simulink model "Vehicle_Validation"  (R2013a)
settings: Solver=ode45  StartTime=0.0  StopTime=10.0  RelTol=1e-3
values from neighbouring files (symbols this model uses):
  Beta = 0    [Vehicle_Val.m]    (also in Vehicle_Val_coastdown.m)
  ks_cmd = .15    (= 0.15)    [Vehicle_Val.m]    (also in Vehicle_Val_coastdown.m)
  Or = 0    [Vehicle_Val.m]    (also in Vehicle_Val_coastdown.m = -0.0157)
  Rc = 10000    [Vehicle_Val.m]    (also in Vehicle_Val_coastdown.m)
  rho = 1.2    [Vehicle_Val.m]    (also in Vehicle_Val_coastdown.m)
  V_cmd = 40    [Vehicle_Val.m]    (also in Vehicle_Val_coastdown.m = 0)
libraries: simulink x2
settings Model: Creator=Nathan  LastModifiedBy=Nathan
settings SolverCC: ZeroCrossControl=DisableAll

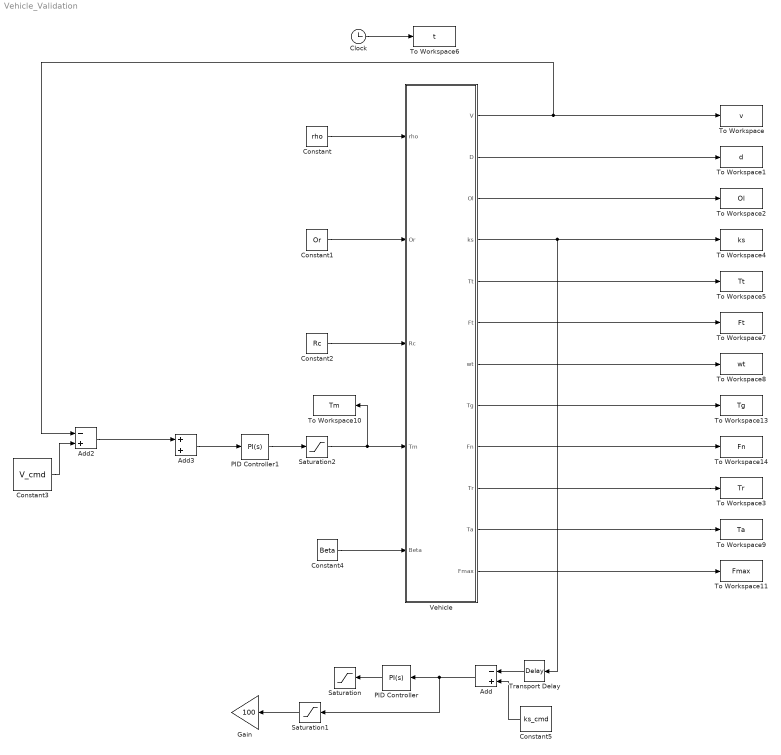
== system Vehicle_Validation ==
  Add : Sum  Inputs=-+
  Add2 : Sum  Inputs=-+
  Add3 : Sum
  Clock : Clock
  Constant : Constant  Value=rho
  Constant1 : Constant  Value=Or
  Constant2 : Constant  Value=Rc
  Constant3 : Constant  Value=V_cmd
  Constant4 : Constant  Value=Beta
  Constant5 : Constant  Value=ks_cmd
  Gain : Gain  Gain=100
  PID Controller : simulink/Continuous/PID Controller  Controller=PI  TimeDomain=Continuous-time  SampleTime=1  IntegratorMethod=Forward Euler  FilterMethod=Forward Euler  Form=Parallel  P=1000  I=5  D=1  N=100  InitialConditionSource=internal  InitialConditionForIntegrator=0  InitialConditionForFilter=0  ExternalReset=none  LimitOutput=off  UpperSaturationLimit=inf  LowerSaturationLimit=-inf  LinearizeAsGain=on  AntiWindupMode=none  Kb=1  TrackingMode=off  Kt=1  PParamMin=[]  PParamMax=[]  IParamMin=[]  IParamMax=[]  DParamMin=[]  DParamMax=[]  NParamMin=[]  NParamMax=[]  KbParamMin=[]  KbParamMax=[]  KtParamMin=[]  KtParamMax=[]  POutMin=[]  POutMax=[]  IOutMin=[]  IOutMax=[]  DOutMin=[]  DOutMax=[]  NOutMin=[]  NOutMax=[]  KbOutMin=[]  KbOutMax=[]  KtOutMin=[]  KtOutMax=[]  IntegratorOutMin=[]  IntegratorOutMax=[]  FilterOutMin=[]  FilterOutMax=[]  SumOutMin=[]  SumOutMax=[]  SumI1OutMin=[]  SumI1OutMax=[]  SumI2OutMin=[]  SumI2OutMax=[]  SumI3OutMin=[]  SumI3OutMax=[]  SumDOutMin=[]  SumDOutMax=[]  SaturationOutMin=[]  SaturationOutMax=[]  IntegratorContinuousStateAttributes=''  IntegratorStateMustResolveToSignalObject=off  IntegratorRTWStateStorageClass=Auto  FilterContinuousStateAttributes=''  FilterStateMustResolveToSignalObject=off  FilterRTWStateStorageClass=Auto
  PID Controller1 : simulink/Continuous/PID Controller  Controller=PI  TimeDomain=Continuous-time  SampleTime=1  IntegratorMethod=Forward Euler  FilterMethod=Forward Euler  Form=Parallel  P=30  I=20  D=1  N=100  InitialConditionSource=internal  InitialConditionForIntegrator=0  InitialConditionForFilter=0  ExternalReset=none  LimitOutput=off  UpperSaturationLimit=inf  LowerSaturationLimit=-inf  LinearizeAsGain=on  AntiWindupMode=none  Kb=1  TrackingMode=off  Kt=1  PParamMin=[]  PParamMax=[]  IParamMin=[]  IParamMax=[]  DParamMin=[]  DParamMax=[]  NParamMin=[]  NParamMax=[]  KbParamMin=[]  KbParamMax=[]  KtParamMin=[]  KtParamMax=[]  POutMin=[]  POutMax=[]  IOutMin=[]  IOutMax=[]  DOutMin=[]  DOutMax=[]  NOutMin=[]  NOutMax=[]  KbOutMin=[]  KbOutMax=[]  KtOutMin=[]  KtOutMax=[]  IntegratorOutMin=[]  IntegratorOutMax=[]  FilterOutMin=[]  FilterOutMax=[]  SumOutMin=[]  SumOutMax=[]  SumI1OutMin=[]  SumI1OutMax=[]  SumI2OutMin=[]  SumI2OutMax=[]  SumI3OutMin=[]  SumI3OutMax=[]  SumDOutMin=[]  SumDOutMax=[]  SaturationOutMin=[]  SaturationOutMax=[]  IntegratorContinuousStateAttributes=''  IntegratorStateMustResolveToSignalObject=off  IntegratorRTWStateStorageClass=Auto  FilterContinuousStateAttributes=''  FilterStateMustResolveToSignalObject=off  FilterRTWStateStorageClass=Auto
  Saturation : Saturate  UpperLimit=0  LowerLimit=-inf
  Saturation1 : Saturate  UpperLimit=0  LowerLimit=-inf
  Saturation2 : Saturate  UpperLimit=inf  LowerLimit=0
  To Workspace : ToWorkspace  VariableName=v  SampleTime=-1
  To Workspace1 : ToWorkspace  VariableName=d  SampleTime=-1
  To Workspace10 : ToWorkspace  VariableName=Tm  SampleTime=-1
  To Workspace11 : ToWorkspace  VariableName=Fmax  SampleTime=-1
  To Workspace13 : ToWorkspace  VariableName=Tg  SampleTime=-1
  To Workspace14 : ToWorkspace  VariableName=Fn  SampleTime=-1
  To Workspace2 : ToWorkspace  VariableName=Ol  SampleTime=-1
  To Workspace3 : ToWorkspace  VariableName=Tr  SampleTime=-1
  To Workspace4 : ToWorkspace  VariableName=ks  SampleTime=-1
  To Workspace5 : ToWorkspace  VariableName=Tt  SampleTime=-1
  To Workspace6 : ToWorkspace  VariableName=t  SampleTime=-1
  To Workspace7 : ToWorkspace  VariableName=Ft  SampleTime=-1
  To Workspace8 : ToWorkspace  VariableName=wt  SampleTime=-1
  To Workspace9 : ToWorkspace  VariableName=Ta  SampleTime=-1
  Transport Delay : TransportDelay  DelayTime=.001
  Vehicle : Subsystem
  wires:
  Constant/1 -> Vehicle/1(rho)
  Constant1/1 -> Vehicle/2(Or)
  Constant2/1 -> Vehicle/3(Rc)
  Constant4/1 -> Vehicle/5(Beta)
  Clock/1 -> To Workspace6/1
  Vehicle/1(V) -> Add2/1, To Workspace/1
  Vehicle/2(D) -> To Workspace1/1
  Vehicle/3(Ol) -> To Workspace2/1
  Vehicle/4(ks) -> Transport Delay/1, To Workspace4/1
  Vehicle/5(Tt) -> To Workspace5/1
  Vehicle/6(Ft) -> To Workspace7/1
  Vehicle/7(wt) -> To Workspace8/1
  Vehicle/8(Tg) -> To Workspace13/1
  Vehicle/9(Fn) -> To Workspace14/1
  Vehicle/10(Tr) -> To Workspace3/1
  Vehicle/11(Ta) -> To Workspace9/1
  Vehicle/12("Fmax ") -> To Workspace11/1
  Add/1 -> Saturation1/1, PID Controller/1
  Constant5/1 -> Add/2
  PID Controller/1 -> Saturation/1
  Constant3/1 -> Add2/2
  Add2/1 -> Add3/1
  Transport Delay/1 -> Add/1
  PID Controller1/1 -> Saturation2/1
  Add3/1 -> PID Controller1/1
  Saturation1/1 -> Gain/1
  Saturation2/1 -> To Workspace10/1, Vehicle/4(Tm)

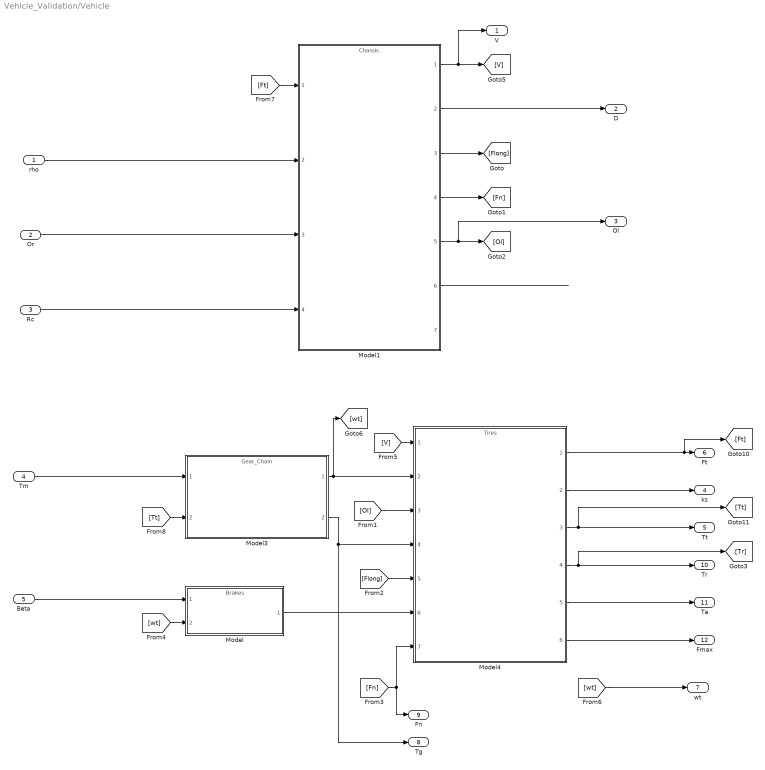
== system Vehicle_Validation/Vehicle ==
  rho : Inport
  Or : Inport  Port=2
  Rc : Inport  Port=3
  Tm : Inport  Port=4
  Beta : Inport  Port=5
  Model : ModelReference  ModelNameDialog=Brakes.slx  SimulationMode=Normal  ModelReferenceVersion=1.3  CopyOfModelName=Brakes.slx  DefaultDataLogging=on
  Model1 : ModelReference  ModelNameDialog=Chassis.slx  SimulationMode=Normal  ModelReferenceVersion=1.14  CopyOfModelName=Chassis.slx  DefaultDataLogging=on
  Model3 : ModelReference  ModelNameDialog=Gear_Chain.slx  SimulationMode=Normal  ModelReferenceVersion=1.13  CopyOfModelName=Gear_Chain.slx  DefaultDataLogging=on
  Model4 : ModelReference  ModelNameDialog=Tires.slx  SimulationMode=Normal  ModelReferenceVersion=1.73  CopyOfModelName=Tires.slx  DefaultDataLogging=on
  V : Outport
  D : Outport  Port=2
  Ol : Outport  Port=3
  ks : Outport  Port=4
  Tt : Outport  Port=5
  Ft : Outport  Port=6
  wt : Outport  Port=7
  Tg : Outport  Port=8
  Fn : Outport  Port=9
  Tr : Outport  Port=10
  Ta : Outport  Port=11
  "Fmax " : Outport  Port=12
  wires:
  Model1/3 -> [Flong]
  [Ol] -> Model4/3
  Model1/4 -> [Fn]
  Model1/5 -> Ol/1, [Ol]
  Model3/1 -> Model4/2, [wt]
  [Tt] -> Model3/2
  [Ft] -> Model1/1
  Model3/2 -> Tg/1, Model4/4
  [wt] -> Model/2
  [V] -> Model4/1
  [Fn] -> Model4/7, Fn/1
  Model1/1 -> V/1, [V]
  [Flong] -> Model4/5
  Model1/6 -> ?
  Or/1 -> Model1/3
  Beta/1 -> Model/1
  Tm/1 -> Model3/1
  Rc/1 -> Model1/4
  rho/1 -> Model1/2
  Model4/1 -> Ft/1, [Ft]
  [wt] -> wt/1
  Model/1 -> Model4/6
  Model1/2 -> D/1
  Model4/2 -> ks/1
  Model4/3 -> [Tt], Tt/1
  Model4/4 -> [Tr], Tr/1
  Model4/5 -> Ta/1
  Model4/6 -> "Fmax "/1
